simulink model "final"  (R2016b)
settings: Solver=VariableStepAuto  StartTime=0.0  StopTime=10.0  RelTol=1e-3
undefined symbols (not defined in the file or in its folder): Capacitor, Start
libraries: powerlib x3
settings Model: Creator=Chandan  LastModifiedBy=Chandan

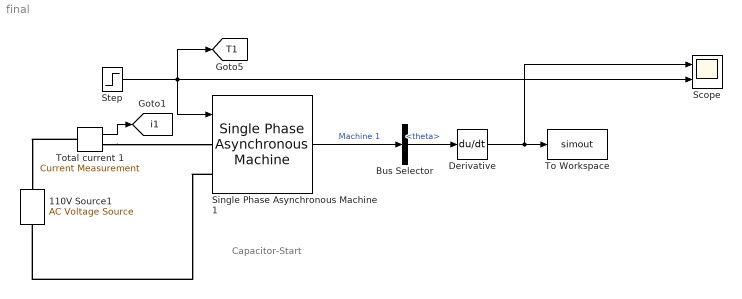
== system final ==
  note: Capacitor-Start
  110V Source1 : powerlib/Electrical Sources/AC Voltage Source  Amplitude=110*sqrt(2)  Phase=90  Frequency=60  SampleTime=0  Measurements=Voltage  BusType=swing  Pref=10e3  Qref=0  Qmin=-inf  Qmax=+inf
  Bus Selector : BusSelector  OutputSignals=theta
  Derivative : Derivative
  Scope : Scope  NumInputPorts=2
  Single Phase Asynchronous Machine 1 : powerlib/Machines/Single Phase Asynchronous Machine  MechanicalLoad=Torque Tm  UNITS=SI  MachineType=Capacitor-Start  MeasurementBus=on  NominalParameters="[ .25*746  110  60]"  MainWindingStator="[2.02  7.4e-3]"  MainWindingRotor="[4.12  5.6e-3]"  MutualInductance=0.177  AuxiliaryWinding=[7.14 8.54e-3]  Mechanical=[0.0146 0 2 1.18]  CapacitorStart="[2.15  255e-6]"  CapacitorRun=[0.04624 1592]  DisconnectionSpeed=75  InitialSpeed=0  DataType=SI  TsPowergui=0  TsBlock=-1
  Step : Step  Time=2  SampleTime=0
  To Workspace : ToWorkspace  VariableName=simout  SaveFormat=Timeseries  SampleTime=-1
  Total current 1 : powerlib/Measurements/Current Measurement  PhasorSimulation=off  OutputType=Complex  PSBequivalent=0
  tag scope: T1=global, i1=global
  wires:
  Bus Selector/1 -> Derivative/1  "<theta>"
  Step/1 -> Scope/2, Single Phase Asynchronous Machine 1/1, [T1]
  Single Phase Asynchronous Machine 1/1 -> Bus Selector/1  "Machine 1"
  Total current 1/1 -> [i1]
  Derivative/1 -> Scope/1, To Workspace/1
  connections:
  Single Phase Asynchronous Machine 1/LConn2 -- 110V Source1/LConn1
  Total current 1/RConn1 -- Single Phase Asynchronous Machine 1/LConn1
  Total current 1/LConn1 -- 110V Source1/RConn1
